simulink model "sampleModel1625"  (R2023a)
settings: Solver=VariableStepAuto  StartTime=0.0  StopTime=10.0  RelTol=1e-3
libraries: hdlsllib x6, simulink x3
settings Model: Creator=user1  LastModifiedBy=user1

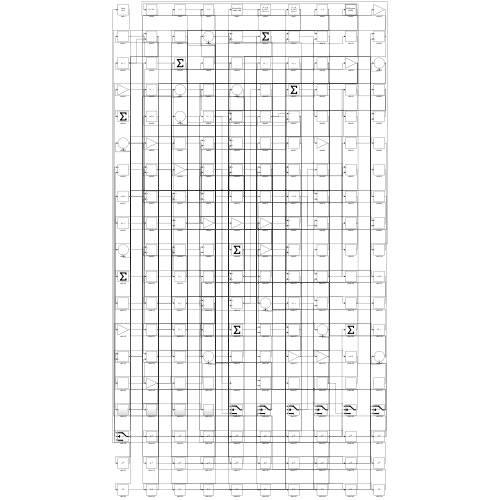
[thumbnail: Simulink's stored preview of the top-level diagram]
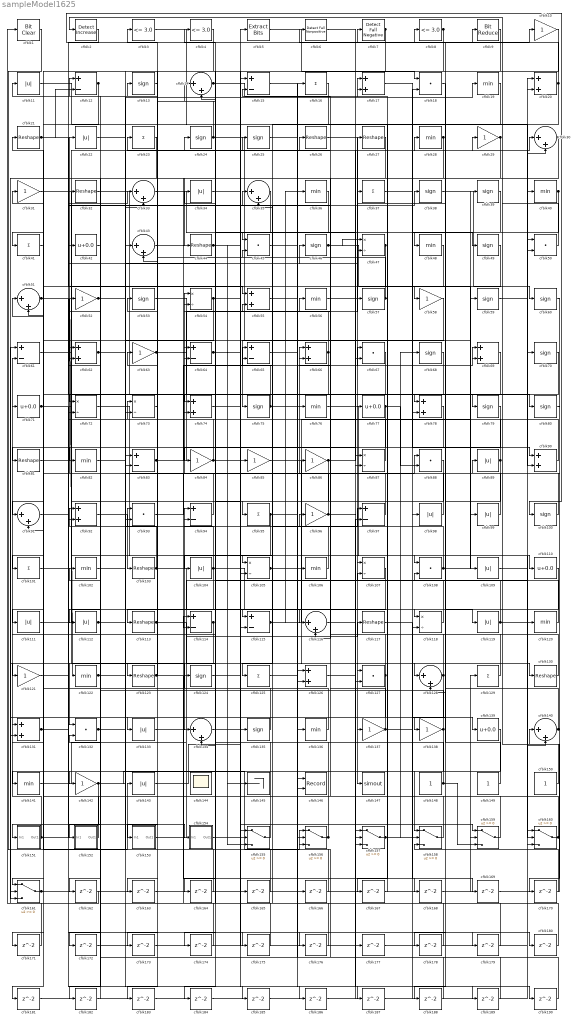
== system sampleModel1625 ==
  cfblk1 : simulink/Logic and Bit Operations/Bit Clear  iBit=0
      settings: LibrarySourceBlock=|
      | hdlsllib/Logic and Bit
      | Operations/Bit Clear
  cfblk{10,29,31,52,58,63,84..86,96,121,137..138,142} (14 alike) : Gain
  cfblk{13,24..25,38..39,46,49,53,57,59..60,68,70,75,79..80,100,124,135} (19 alike) : Signum
  cfblk{16,23,37,41,95,101,125,129} (8 alike) : Sum  Inputs=+
  cfblk{19,28,36,40,48,56,76,82,102,106,120,122,136,141} (14 alike) : MinMax
  cfblk{21,26..27,32,44,81,103,113,117,123,130} (11 alike) : Reshape
  cfblk{11,22,34,89,98..99,104,109,111..112,119,133,143} (13 alike) : Abs  SaturateOnIntegerOverflow=off
  cfblk{47,54,72..73,87,105,107,118} (8 alike) : Product  Inputs=*/  RndMeth=Zero  SaturateOnIntegerOverflow=on
  cfblk{18,45,50,67,88,93,108,127,132} (9 alike) : DotProduct  OutDataTypeStr=Inherit: Inherit via internal rule
  cfblk{42,71,77,110,139} (5 alike) : Bias  Bias=0.0  SaturateOnIntegerOverflow=off
  cfblk{12,15,61,64..65,83,94,97,114..115} (10 alike) : Sum  Inputs=+-
  cfblk{14,30,33,35,43,51,91,116,128,134,140} (11 alike) : Sum  Inputs=|++
  cfblk{17,20,55,62,66,69,74,78,90,92,126,131} (12 alike) : Sum
  cfblk144 : Scope
      settings: Floating=on
  cfblk145 : Terminator
  cfblk146 : Record  FileSettingsInternal="{\"entries\":[{\"content\":{\"excelSettings\":{\"content\":{},\"type\":\"Streamout.ExcelSettings\"}},\"type\":\"Streamout.FileSettingStorage\",\"uuid\":\"\"}],\"packageUris\":[\"http:\\/\\/schema.mathworks.com\\/mf0\\/streamout_blocks\\/R2020a\"],\"version\":\"1.0\"}"  Layout=[1 1]  SignalsInternal="{\"entries\":[{\"content\":{\"signals\":[{\"content\":{\"blockPath\":[],\"dimensions\":[1],\"domain\":\"\",\"lineColor\":\"#a2142f\",\"plots\":[1],\"port\":1,\"signalID\":2359,\"signalName\":\"XY Graph:1\"},\"type\":\"RecordBlkView.Signal\",\"uuid\":\"\"},{\"content\":{\"blockPath\":[],\"dimensions\":[1],\"domain\":\"\",\"lineColor\":\"#139fff\",\"plots\":[1],\"port\":2,\"signalID\":2362,\"signalName\":\"XY Graph:2\"},\"type\":\"RecordBlkView.Signal\",\"uuid\":\"\"}]},\"type\":\"RecordBlkView.InputSignals\",\"uuid\":\"\"}],\"packageUris\":[\"http:\\/\\/schema.mathworks.com\\/mf0\\/streamout_blocks\\/R2020a\"],\"version\":\"1.0\"}"  VisualizationBindings="{\"xyplotplugin\":{\"info\":[{\"series\":[{\"bindingParametersList\":[{\"parameter\":\"X-Axis\",\"signalID\":2359,\"signalName\":\"XY Graph:1\"},{\"parameter\":\"Y-Axis\",\"signalID\":2362,\"signalName\":\"XY Graph:2\"}],\"seriesID\":11529}],\"subplotID\":1}]}}"  CompatibilityTag=XY  st=-1
  cfblk147 : ToWorkspace  VariableName=simout  SaveFormat=Timeseries  SampleTime=-1
  cfblk148 : Constant  SampleTime=-1
  cfblk149 : Constant  SampleTime=-1
  cfblk150 : Constant  SampleTime=-1
  cfblk151 : Subsystem
      settings: LibrarySourceBlock=|
      | hdlsllib/Ports &
      | Subsystems/Subsystem
  cfblk152 : Subsystem
      settings: LibrarySourceBlock=|
      | hdlsllib/Ports &
      | Subsystems/Subsystem
  cfblk153 : Subsystem
      settings: LibrarySourceBlock=|
      | hdlsllib/Ports &
      | Subsystems/Subsystem
  cfblk154 : Subsystem
      settings: LibrarySourceBlock=|
      | hdlsllib/Ports &
      | Subsystems/Subsystem
  cfblk{155..161} (7 alike) : Switch  SaturateOnIntegerOverflow=off  InputSameDT=off
  cfblk{162..190} (29 alike) : Delay  SampleTime=1
  cfblk2 : simulink/Logic and Bit Operations/Detect Increase  vinit=0.0  OutDataTypeStr=boolean
      settings: LibrarySourceBlock=|
      | hdlsllib/Logic and Bit
      | Operations/Detect
      | Increase
  cfblk3 : hdlsllib/Logic and Bit Operations/Compare To Constant  relop=<=  const=3.0  OutDataTypeStr=boolean
  cfblk4 : hdlsllib/Logic and Bit Operations/Compare To Constant  relop=<=  const=3.0  OutDataTypeStr=boolean
  cfblk5 : simulink/Logic and Bit Operations/Extract Bits  bitsToExtract=Upper half  numBits=8  bitIdxRange=[0 7]  outScalingMode=Preserve fixed-point scaling
      settings: LibrarySourceBlock=|
      | hdlsllib/Logic and Bit
      | Operations/Extract Bits
  cfblk6 : hdlsllib/Logic and Bit Operations/Detect Fall Nonpositive  vinit=0  OutDataTypeStr=boolean
  cfblk7 : hdlsllib/Logic and Bit Operations/Detect Fall Negative  vinit=0  OutDataTypeStr=boolean
  cfblk8 : hdlsllib/Logic and Bit Operations/Compare To Constant  relop=<=  const=3.0  OutDataTypeStr=boolean
  cfblk9 : hdlsllib/Logic and Bit Operations/Bit Reduce  mode=AND
  wires:
  cfblk31/1 -> cfblk118/1
  cfblk54/1 -> cfblk78/2, cfblk171/1
  cfblk155/1 -> cfblk61/2
  cfblk72/1 -> cfblk108/1
  cfblk58/1 -> cfblk75/1
  cfblk90/1 -> cfblk65/1
  cfblk151/1(Out1) -> cfblk71/1, cfblk33/1, cfblk7/1
  cfblk135/1 -> cfblk94/1
  cfblk28/1 -> cfblk44/1, cfblk116/2
  cfblk38/1 -> cfblk60/1
  cfblk156/1 -> cfblk73/1, cfblk42/1
  cfblk103/1 -> cfblk115/1, cfblk12/1
  cfblk36/1 -> cfblk105/1
  cfblk7/1 -> cfblk113/1, cfblk41/1
  cfblk41/1 -> cfblk101/1
  cfblk111/1 -> cfblk26/1
  cfblk48/1 -> cfblk147/1
  cfblk33/1 -> cfblk157/1
  cfblk44/1 -> cfblk145/1, cfblk176/1
  cfblk4/1 -> cfblk133/1
  cfblk26/1 -> cfblk107/1
  cfblk119/1 -> cfblk120/1, cfblk55/2
  cfblk1/1 -> cfblk143/1
  cfblk149/1 -> cfblk108/2
  cfblk142/1 -> cfblk156/1, cfblk161/1, cfblk33/2
  cfblk53/1 -> cfblk79/1
  cfblk50/1 -> cfblk2/1
  cfblk95/1 -> cfblk146/1, cfblk134/2
  cfblk114/1 -> cfblk132/1, cfblk131/2
  cfblk51/1 -> cfblk122/1, cfblk74/2
  cfblk14/1 -> cfblk17/1, cfblk84/1
  cfblk129/1 -> cfblk8/1
  cfblk93/1 -> cfblk88/1
  cfblk32/1 -> cfblk80/1
  cfblk104/1 -> cfblk146/2, cfblk94/2, cfblk173/1
  cfblk60/1 -> cfblk89/1
  cfblk131/1 -> cfblk38/1, cfblk10/1
  cfblk138/1 -> cfblk158/1, cfblk52/1
  cfblk87/1 -> cfblk22/1
  cfblk8/1 -> cfblk104/1, cfblk174/1
  cfblk136/1 -> cfblk21/1
  cfblk125/1 -> cfblk16/1
  cfblk37/1 -> cfblk90/1
  cfblk97/1 -> cfblk66/1
  cfblk106/1 -> cfblk65/2
  cfblk30/1 -> cfblk123/1, cfblk112/1
  cfblk118/1 -> cfblk24/1
  cfblk5/1 -> cfblk18/1
  cfblk59/1 -> cfblk20/1
  cfblk3/1 -> cfblk70/1
  cfblk45/1 -> cfblk76/1
  cfblk112/1 -> cfblk19/1, cfblk175/1
  cfblk71/1 -> cfblk110/1, cfblk179/1
  cfblk157/1 -> cfblk118/2, cfblk68/1
  cfblk94/1 -> cfblk54/1
  cfblk153/1(Out1) -> cfblk117/1
  cfblk75/1 -> cfblk127/1, cfblk4/1
  cfblk18/1 -> cfblk58/1
  cfblk83/1 -> cfblk27/1, cfblk69/2
  cfblk123/1 -> cfblk93/1, cfblk168/1
  cfblk24/1 -> cfblk99/1, cfblk3/1
  cfblk76/1 -> cfblk160/2
  cfblk137/1 -> cfblk56/1, cfblk139/1
  cfblk85/1 -> cfblk128/1
  cfblk126/1 -> cfblk130/1
  cfblk2/1 -> cfblk100/1
  cfblk132/1 -> cfblk92/1, cfblk46/1
  cfblk100/1 -> cfblk62/1
  cfblk57/1 -> cfblk11/1, cfblk167/1
  cfblk86/1 -> cfblk29/1, cfblk164/1
  cfblk6/1 -> cfblk87/1
  cfblk122/1 -> cfblk97/1, cfblk47/2
  cfblk99/1 -> cfblk35/1
  cfblk56/1 -> cfblk77/1
  cfblk82/1 -> cfblk43/1
  cfblk96/1 -> cfblk13/1, cfblk35/2, cfblk190/1
  cfblk29/1 -> cfblk48/1, cfblk114/2, cfblk161/3, cfblk128/2
  cfblk11/1 -> cfblk90/2
  cfblk84/1 -> cfblk63/1, cfblk69/1
  cfblk108/1 -> cfblk59/1, cfblk66/2
  cfblk81/1 -> cfblk135/1
  cfblk23/1 -> cfblk83/2
  cfblk107/1 -> cfblk153/1(In1)
  cfblk133/1 -> cfblk40/1
  cfblk140/1 -> cfblk107/2, cfblk37/1
  cfblk10/1 -> cfblk105/2
  cfblk115/1 -> cfblk39/1, cfblk36/1
  cfblk89/1 -> cfblk34/1, cfblk188/1
  cfblk154/1(Out1) -> cfblk67/1
  cfblk134/1 -> cfblk57/1
  cfblk42/1 -> cfblk72/1
  cfblk43/1 -> cfblk119/1
  cfblk98/1 -> cfblk31/1
  cfblk139/1 -> cfblk155/2
  cfblk49/1 -> cfblk138/1
  cfblk64/1 -> cfblk159/1, cfblk155/3
  cfblk79/1 -> cfblk157/3
  cfblk141/1 -> cfblk98/1
  cfblk158/1 -> cfblk96/1
  cfblk27/1 -> cfblk142/1
  cfblk91/1 -> cfblk154/1(In1)
  cfblk92/1 -> cfblk103/1
  cfblk20/1 -> cfblk125/1, cfblk6/1
  cfblk40/1 -> cfblk78/1, cfblk115/2
  cfblk120/1 -> cfblk64/1
  cfblk9/1 -> cfblk73/2
  cfblk47/1 -> cfblk93/2, cfblk121/1
  cfblk69/1 -> cfblk81/1
  cfblk101/1 -> cfblk134/1
  cfblk17/1 -> cfblk49/1
  cfblk143/1 -> cfblk5/1
  cfblk148/1 -> cfblk141/1, cfblk54/2, cfblk159/3
  cfblk161/1 -> cfblk140/1, cfblk129/1
  cfblk21/1 -> cfblk55/1, cfblk12/2
  cfblk39/1 -> cfblk124/1
  cfblk152/1(Out1) -> cfblk131/1
  cfblk159/1 -> cfblk102/1
  cfblk66/1 -> cfblk14/2, cfblk82/1, cfblk91/1
  cfblk77/1 -> cfblk111/1, cfblk88/2
  cfblk128/1 -> cfblk32/1, cfblk161/2
  cfblk35/1 -> cfblk74/1
  cfblk12/1 -> cfblk151/1(In1), cfblk91/2
  cfblk13/1 -> cfblk43/2
  cfblk150/1 -> cfblk9/1
  cfblk113/1 -> cfblk140/2, cfblk53/1, cfblk183/1
  cfblk102/1 -> cfblk86/1
  cfblk127/1 -> cfblk15/2, cfblk162/1
  cfblk15/1 -> cfblk126/2
  cfblk88/1 -> cfblk95/1
  cfblk130/1 -> cfblk23/1
  cfblk62/1 -> cfblk25/1, cfblk185/1
  cfblk16/1 -> cfblk45/1
  cfblk25/1 -> cfblk106/1
  cfblk19/1 -> cfblk137/1
  cfblk63/1 -> cfblk136/1, cfblk87/2
  cfblk46/1 -> cfblk109/1, cfblk47/1
  cfblk61/1 -> cfblk85/1
  cfblk160/1 -> cfblk51/2, cfblk62/2
  cfblk22/1 -> cfblk67/2
  cfblk52/1 -> cfblk152/1(In1), cfblk116/1
  cfblk105/1 -> cfblk30/1, cfblk28/1
  cfblk109/1 -> cfblk50/1
  cfblk162/1 -> cfblk1/1
  cfblk73/1 -> cfblk163/1
  cfblk163/1 -> cfblk127/2
  cfblk164/1 -> cfblk83/1
  cfblk124/1 -> cfblk165/1
  cfblk165/1 -> cfblk14/1
  cfblk65/1 -> cfblk166/1
  cfblk166/1 -> cfblk51/1
  cfblk167/1 -> cfblk17/2
  cfblk168/1 -> cfblk159/2
  cfblk117/1 -> cfblk169/1
  cfblk169/1 -> cfblk160/1
  cfblk80/1 -> cfblk170/1
  cfblk170/1 -> cfblk158/3
  cfblk171/1 -> cfblk61/1
  cfblk78/1 -> cfblk172/1
  cfblk172/1 -> cfblk155/1
  cfblk173/1 -> cfblk30/2
  cfblk174/1 -> cfblk114/1
  cfblk175/1 -> cfblk64/2
  cfblk176/1 -> cfblk126/1
  cfblk116/1 -> cfblk177/1
  cfblk177/1 -> cfblk20/2
  cfblk110/1 -> cfblk178/1
  cfblk178/1 -> cfblk132/2
  cfblk179/1 -> cfblk45/2
  cfblk74/1 -> cfblk180/1
  cfblk180/1 -> cfblk15/1
  cfblk70/1 -> cfblk181/1
  cfblk181/1 -> cfblk157/2
  cfblk68/1 -> cfblk182/1
  cfblk182/1 -> cfblk92/2
  cfblk183/1 -> cfblk97/2
  cfblk67/1 -> cfblk184/1
  cfblk184/1 -> cfblk160/3
  cfblk185/1 -> cfblk50/2
  cfblk121/1 -> cfblk186/1
  cfblk186/1 -> cfblk18/2
  cfblk34/1 -> cfblk187/1
  cfblk187/1 -> cfblk158/2
  cfblk188/1 -> cfblk156/2
  cfblk55/1 -> cfblk189/1
  cfblk189/1 -> cfblk72/2
  cfblk190/1 -> cfblk156/3

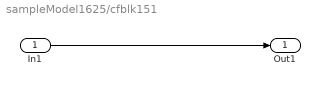
== system sampleModel1625/cfblk151 ==
  In1 : Inport
  Out1 : Outport
  wires:
  In1/1 -> Out1/1

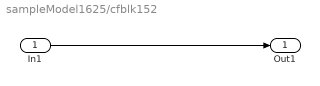
== system sampleModel1625/cfblk152 ==
  In1 : Inport
  Out1 : Outport
  wires:
  In1/1 -> Out1/1

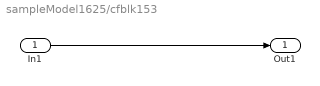
== system sampleModel1625/cfblk153 ==
  In1 : Inport
  Out1 : Outport
  wires:
  In1/1 -> Out1/1

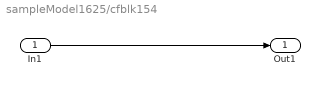
== system sampleModel1625/cfblk154 ==
  In1 : Inport
  Out1 : Outport
  wires:
  In1/1 -> Out1/1
